simulink model "simulinkTest"  (R2015b)
settings: Solver=FixedStepDiscrete  StartTime=0.0  StopTime=10.0  FixedStep=1/5000  RelTol=1e-3
libraries: MegaNeurOne x1
settings Model: Creator=BCI2000  LastModifiedBy=BCI2000

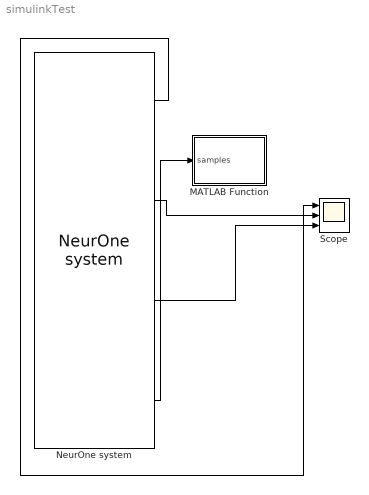
== system simulinkTest ==
  MATLAB Function : MATLAB Function  TreatAsAtomicUnit=on
  NeurOne system : MegaNeurOne/NeurOne system  Description=This block drives an online measurement in a NeurOne system.  strDrvDataPath=C:\ProgramData\Mega Electronics Ltd\NeurOne64  strSimuFilePath=E:\NeurOne\NeurOneUser\HaWeNBD7\test.sdn  cbxSampleRate=5000  vecInpNums=1:77  vecInpModes=zeros(77)  strDevFilterName=LP __1250 Hz (80 kHz_5000 Hz)  edtFrameSize=500
      settings: AttributesFormatString=|
      | Fs=%<cbxSamplerate> Hz
      | Double-click to configure
  Scope : Scope  NumInputPorts=3
  wires:
  NeurOne system/1 -> Scope/1
  NeurOne system/2 -> Scope/2
  NeurOne system/3 -> Scope/3
  NeurOne system/4 -> MATLAB Function/1(samples)

== matlab function simulinkTest/MATLAB Function ==
  data: samples input
function displaySampleSize(samples)
%#codegen
fprintf('x:%f y:%f',size(samples,1),size(samples,2));
